simulink model "sampleModel1797"  (R2023a)
settings: Solver=VariableStepAuto  StartTime=0.0  StopTime=10.0  RelTol=1e-3
libraries: hdlsllib x7, simulink x3
settings Model: Creator=user1  LastModifiedBy=user1

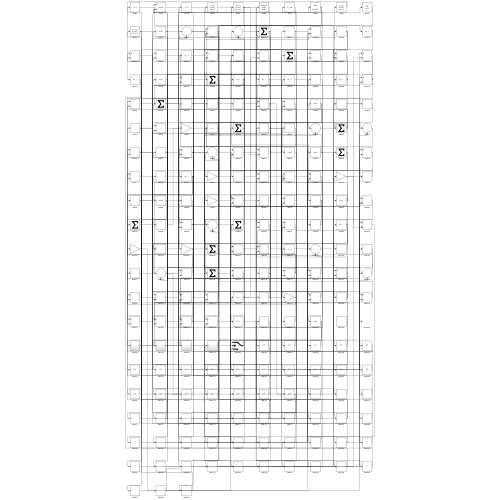
[thumbnail: Simulink's stored preview of the top-level diagram]
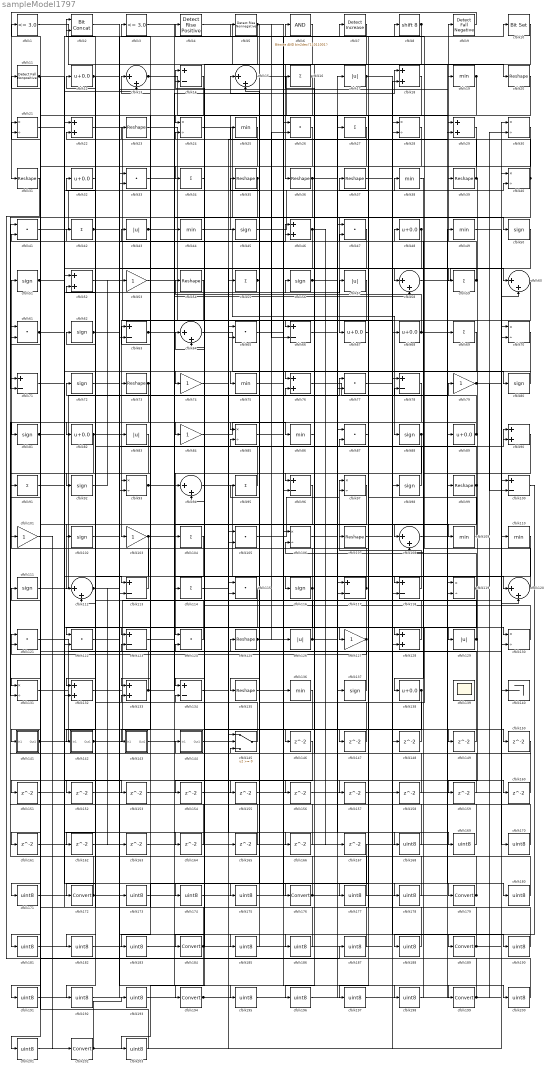
== system sampleModel1797 ==
  cfblk1 : hdlsllib/Logic and Bit Operations/Compare To Constant  relop=<=  const=3.0  OutDataTypeStr=boolean
  cfblk10 : simulink/Logic and Bit Operations/Bit Set  iBit=0
      settings: LibrarySourceBlock=|
      | hdlsllib/Logic and Bit
      | Operations/Bit Set
  cfblk{14,63,66,71,78,96,100,113,117..118,123,134} (12 alike) : Sum  Inputs=+-
  cfblk{53,74,79,84,101,103,127} (7 alike) : Gain
  cfblk{45,50..51,56,62,72,80..81,88,92,98,102,111,116,137} (15 alike) : Signum
  cfblk{16,27,34,42,55,59,69,91,95,104,114} (11 alike) : Sum  Inputs=+
  cfblk{26,33,41,47,61,65,77,87,105,115,121..122,124} (13 alike) : DotProduct  OutDataTypeStr=Inherit: Inherit via internal rule
  cfblk{21,24,28,30,40,70,85,93,97,106,119,130..131} (13 alike) : Product  Inputs=*/  RndMeth=Zero  SaturateOnIntegerOverflow=on
  cfblk{20,23,31,35..37,39,54,73,99,107,125,135} (13 alike) : Reshape
  cfblk{13,15,58,60,64,94,108,112,120} (9 alike) : Sum  Inputs=|++
  cfblk{19,25,38,44,49,75,86,109..110,136} (10 alike) : MinMax
  cfblk11 : hdlsllib/Logic and Bit Operations/Detect Fall Nonpositive  vinit=0  OutDataTypeStr=boolean
  cfblk{12,32,48,67..68,82,89,138} (8 alike) : Bias  Bias=0.0  SaturateOnIntegerOverflow=off
  cfblk{17,43,57,83,126,129} (6 alike) : Abs  SaturateOnIntegerOverflow=off
  cfblk{18,22,29,46,52,76,90,128,132..133} (10 alike) : Sum
  cfblk139 : Scope
      settings: Floating=on
  cfblk140 : Terminator
  cfblk141 : Subsystem
      settings: LibrarySourceBlock=|
      | hdlsllib/Ports &
      | Subsystems/Subsystem
  cfblk142 : Subsystem
      settings: LibrarySourceBlock=|
      | hdlsllib/Ports &
      | Subsystems/Subsystem
  cfblk143 : Subsystem
      settings: LibrarySourceBlock=|
      | hdlsllib/Ports &
      | Subsystems/Subsystem
  cfblk144 : Subsystem
      settings: LibrarySourceBlock=|
      | hdlsllib/Ports &
      | Subsystems/Subsystem
  cfblk145 : Switch  SaturateOnIntegerOverflow=off  InputSameDT=off
  cfblk{146..167} (22 alike) : Delay  SampleTime=1
  cfblk{168..171,173..175,177..178,180..183,185..188,190..193,195..198,200..201,203} (28 alike) : DataTypeConversion  OutDataTypeStr=uint8  SaturateOnIntegerOverflow=off  RndMeth=Floor
  cfblk{172,176,179,184,189,194,199,202} (8 alike) : DataTypeConversion  SaturateOnIntegerOverflow=off  RndMeth=Floor
  cfblk2 : hdlsllib/Logic and Bit Operations/Bit Concat  numInputs=2
  cfblk3 : hdlsllib/Logic and Bit Operations/Compare To Constant  relop=<=  const=3.0  OutDataTypeStr=boolean
  cfblk4 : hdlsllib/Logic and Bit Operations/Detect Rise Positive  vinit=0  OutDataTypeStr=boolean
  cfblk5 : hdlsllib/Logic and Bit Operations/Detect Rise Nonnegative  vinit=0  OutDataTypeStr=boolean
  cfblk6 : simulink/Logic and Bit Operations/Bitwise Operator  logicop=AND  UseBitMask=on  BitMask=bin2dec('11011001')  BitMaskRealWorld=Stored Integer
      settings: LibrarySourceBlock=|
      | hdlsllib/Logic and Bit
      | Operations/Bitwise
      | Operator
  cfblk7 : simulink/Logic and Bit Operations/Detect Increase  vinit=0.0  OutDataTypeStr=boolean
      settings: LibrarySourceBlock=|
      | hdlsllib/Logic and Bit
      | Operations/Detect
      | Increase
  cfblk8 : ArithShift  BitShiftNumber=8
  cfblk9 : hdlsllib/Logic and Bit Operations/Detect Fall Negative  vinit=0  OutDataTypeStr=boolean
  wires:
  cfblk22/1 -> cfblk66/1
  cfblk44/1 -> cfblk88/1
  cfblk27/1 -> cfblk172/1
  cfblk38/1 -> cfblk122/1
  cfblk94/1 -> cfblk116/1
  cfblk121/1 -> cfblk125/1
  cfblk127/1 -> cfblk121/1, cfblk2/1
  cfblk120/1 -> cfblk4/1
  cfblk138/1 -> cfblk154/1, cfblk155/1
  cfblk113/1 -> cfblk51/1
  cfblk57/1 -> cfblk103/1
  cfblk9/1 -> cfblk31/1
  cfblk92/1 -> cfblk53/1
  cfblk5/1 -> cfblk74/1, cfblk130/1, cfblk66/2, cfblk175/1
  cfblk23/1 -> cfblk98/1
  cfblk19/1 -> cfblk45/1, cfblk29/2
  cfblk105/1 -> cfblk97/1
  cfblk20/1 -> cfblk24/1
  cfblk124/1 -> cfblk63/1
  cfblk69/1 -> cfblk194/1
  cfblk90/1 -> cfblk138/1
  cfblk47/1 -> cfblk176/1
  cfblk34/1 -> cfblk134/1
  cfblk118/1 -> cfblk97/2
  cfblk145/1 -> cfblk72/1
  cfblk109/1 -> cfblk37/1
  cfblk58/1 -> cfblk60/1
  cfblk8/1 -> cfblk76/1, cfblk96/2
  cfblk119/1 -> cfblk135/1, cfblk106/2
  cfblk64/1 -> cfblk80/1
  cfblk111/1 -> cfblk77/1
  cfblk36/1 -> cfblk109/1, cfblk141/1(In1)
  cfblk63/1 -> cfblk120/1, cfblk198/1
  cfblk89/1 -> cfblk12/1, cfblk81/1
  cfblk61/1 -> cfblk13/2, cfblk153/1
  cfblk126/1 -> cfblk87/1, cfblk2/2
  cfblk24/1 -> cfblk67/1
  cfblk80/1 -> cfblk75/1
  cfblk141/1(Out1) -> cfblk70/2, cfblk149/1
  cfblk131/1 -> cfblk44/1
  cfblk4/1 -> cfblk36/1
  cfblk10/1 -> cfblk84/1
  cfblk11/1 -> cfblk127/1, cfblk131/1
  cfblk82/1 -> cfblk121/2, cfblk90/2
  cfblk84/1 -> cfblk86/1
  cfblk104/1 -> cfblk132/1
  cfblk76/1 -> cfblk79/1
  cfblk71/1 -> cfblk113/1
  cfblk32/1 -> cfblk82/1
  cfblk95/1 -> cfblk62/1
  cfblk101/1 -> cfblk202/1
  cfblk125/1 -> cfblk26/1, cfblk26/2
  cfblk142/1(Out1) -> cfblk55/1, cfblk56/1
  cfblk99/1 -> cfblk15/2, cfblk108/2, cfblk147/1
  cfblk117/1 -> cfblk95/1, cfblk24/2
  cfblk14/1 -> cfblk93/1
  cfblk88/1 -> cfblk124/1, cfblk85/2
  cfblk30/1 -> cfblk94/1
  cfblk13/1 -> cfblk89/1, cfblk58/1
  cfblk17/1 -> cfblk73/1, cfblk190/1
  cfblk33/1 -> cfblk189/1
  cfblk59/1 -> cfblk9/1, cfblk21/1
  cfblk133/1 -> cfblk40/2, cfblk21/2
  cfblk106/1 -> cfblk90/1
  cfblk65/1 -> cfblk199/1
  cfblk62/1 -> cfblk46/2, cfblk182/1
  cfblk91/1 -> cfblk179/1
  cfblk112/1 -> cfblk6/1, cfblk163/1
  cfblk1/1 -> cfblk119/1
  cfblk41/1 -> cfblk17/1
  cfblk45/1 -> cfblk39/1
  cfblk129/1 -> cfblk48/1, cfblk16/1
  cfblk87/1 -> cfblk7/1
  cfblk81/1 -> cfblk57/1, cfblk38/1
  cfblk35/1 -> cfblk92/1, cfblk122/2
  cfblk86/1 -> cfblk46/1
  cfblk2/1 -> cfblk83/1
  cfblk42/1 -> cfblk19/1, cfblk5/1
  cfblk51/1 -> cfblk8/1, cfblk59/1
  cfblk137/1 -> cfblk23/1
  cfblk96/1 -> cfblk112/1
  cfblk48/1 -> cfblk93/2, cfblk114/1
  cfblk12/1 -> cfblk20/1, cfblk162/1
  cfblk130/1 -> cfblk14/1
  cfblk132/1 -> cfblk60/2
  cfblk93/1 -> cfblk118/1, cfblk58/2
  cfblk50/1 -> cfblk105/2
  cfblk39/1 -> cfblk14/2, cfblk159/1
  cfblk98/1 -> cfblk64/2
  cfblk114/1 -> cfblk87/2
  cfblk6/1 -> cfblk104/1
  cfblk128/1 -> cfblk42/1
  cfblk46/1 -> cfblk143/1(In1), cfblk167/1
  cfblk73/1 -> cfblk123/1, cfblk131/2, cfblk171/1
  cfblk70/1 -> cfblk132/2
  cfblk116/1 -> cfblk142/1(In1), cfblk11/1
  cfblk102/1 -> cfblk63/2
  cfblk54/1 -> cfblk133/1
  cfblk7/1 -> cfblk34/1
  cfblk26/1 -> cfblk102/1
  cfblk56/1 -> cfblk129/1, cfblk128/1
  cfblk103/1 -> cfblk112/2, cfblk18/1
  cfblk15/1 -> cfblk137/1
  cfblk79/1 -> cfblk140/1, cfblk100/2
  cfblk53/1 -> cfblk117/2
  cfblk75/1 -> cfblk10/1
  cfblk43/1 -> cfblk50/1, cfblk108/1
  cfblk77/1 -> cfblk118/2
  cfblk40/1 -> cfblk22/2, cfblk71/2
  cfblk25/1 -> cfblk184/1
  cfblk16/1 -> cfblk96/1, cfblk191/1
  cfblk134/1 -> cfblk29/1
  cfblk115/1 -> cfblk145/2
  cfblk68/1 -> cfblk54/1, cfblk150/1
  cfblk55/1 -> cfblk35/1, cfblk85/1
  cfblk60/1 -> cfblk146/1
  cfblk147/1 -> cfblk117/1
  cfblk37/1 -> cfblk148/1
  cfblk148/1 -> cfblk15/1
  cfblk149/1 -> cfblk94/2
  cfblk150/1 -> cfblk145/3
  cfblk97/1 -> cfblk151/1
  cfblk151/1 -> cfblk22/1
  cfblk29/1 -> cfblk152/1
  cfblk152/1 -> cfblk145/1
  cfblk153/1 -> cfblk100/1
  cfblk154/1 -> cfblk64/1
  cfblk123/1 -> cfblk156/1
  cfblk156/1 -> cfblk30/1
  cfblk85/1 -> cfblk157/1
  cfblk157/1 -> cfblk40/1
  cfblk107/1 -> cfblk158/1
  cfblk158/1 -> cfblk61/1
  cfblk159/1 -> cfblk76/2
  cfblk74/1 -> cfblk160/1
  cfblk160/1 -> cfblk13/1
  cfblk83/1 -> cfblk161/1
  cfblk161/1 -> cfblk119/2
  cfblk162/1 -> cfblk113/2
  cfblk163/1 -> cfblk133/2
  cfblk21/1 -> cfblk164/1
  cfblk164/1 -> cfblk71/1
  cfblk165/1 -> cfblk115/1
  cfblk144/1(Out1) -> cfblk166/1
  cfblk166/1 -> cfblk1/1
  cfblk3/1 -> cfblk168/1
  cfblk168/1 -> cfblk43/1
  cfblk66/1 -> cfblk169/1
  cfblk169/1 -> cfblk3/1
  cfblk49/1 -> cfblk170/1
  cfblk170/1 -> cfblk105/1
  cfblk171/1 -> cfblk49/1
  cfblk172/1 -> cfblk41/2, cfblk32/1
  cfblk122/1 -> cfblk173/1
  cfblk173/1 -> cfblk27/1
  cfblk136/1 -> cfblk174/1
  cfblk174/1 -> cfblk126/1
  cfblk175/1 -> cfblk136/1
  cfblk176/1 -> cfblk128/2, cfblk41/1, cfblk106/1
  cfblk67/1 -> cfblk177/1
  cfblk177/1 -> cfblk47/1
  cfblk155/1 -> cfblk178/1
  cfblk178/1 -> cfblk47/2
  cfblk179/1 -> cfblk124/2, cfblk134/2
  cfblk108/1 -> cfblk180/1
  cfblk180/1 -> cfblk91/1
  cfblk28/1 -> cfblk181/1
  cfblk181/1 -> cfblk115/2
  cfblk182/1 -> cfblk28/1
  cfblk167/1 -> cfblk183/1
  cfblk183/1 -> cfblk28/2
  cfblk184/1 -> cfblk18/2, cfblk144/1(In1), cfblk123/2, cfblk203/1
  cfblk143/1(Out1) -> cfblk185/1
  cfblk185/1 -> cfblk25/1
  cfblk52/1 -> cfblk186/1
  cfblk186/1 -> cfblk61/2
  cfblk31/1 -> cfblk187/1
  cfblk187/1 -> cfblk52/1
  cfblk100/1 -> cfblk188/1
  cfblk188/1 -> cfblk52/2
  cfblk189/1 -> cfblk130/2, cfblk107/1
  cfblk190/1 -> cfblk33/1
  cfblk191/1 -> cfblk33/2
  cfblk110/1 -> cfblk192/1
  cfblk192/1 -> cfblk165/1
  cfblk193/1 -> cfblk110/1
  cfblk194/1 -> cfblk99/1, cfblk70/1
  cfblk72/1 -> cfblk195/1
  cfblk195/1 -> cfblk69/1
  cfblk78/1 -> cfblk196/1
  cfblk196/1 -> cfblk77/2
  cfblk18/1 -> cfblk197/1
  cfblk197/1 -> cfblk78/1
  cfblk198/1 -> cfblk78/2
  cfblk199/1 -> cfblk111/1, cfblk30/2
  cfblk135/1 -> cfblk200/1
  cfblk200/1 -> cfblk65/1
  cfblk146/1 -> cfblk201/1
  cfblk201/1 -> cfblk65/2
  cfblk202/1 -> cfblk193/1, cfblk68/1, cfblk120/2
  cfblk203/1 -> cfblk101/1

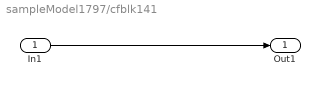
== system sampleModel1797/cfblk141 ==
  In1 : Inport
  Out1 : Outport
  wires:
  In1/1 -> Out1/1

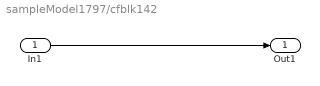
== system sampleModel1797/cfblk142 ==
  In1 : Inport
  Out1 : Outport
  wires:
  In1/1 -> Out1/1

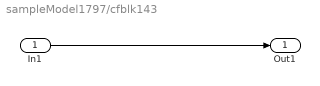
== system sampleModel1797/cfblk143 ==
  In1 : Inport
  Out1 : Outport
  wires:
  In1/1 -> Out1/1

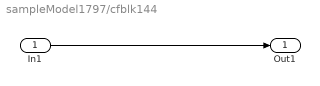
== system sampleModel1797/cfblk144 ==
  In1 : Inport
  Out1 : Outport
  wires:
  In1/1 -> Out1/1
